simulink model "Team_Fire_Simulink_Model_Final_Presantation"  (R2025a)
settings: Solver=VariableStepAuto  StartTime=0.0  StopTime=12  RelTol=1e-3
libraries: spsControlledVoltageSourceLib x1, spsDCMachineLib x1, fl_lib x1, simulink x1, SignalEditorBlockLib x1, sps_lib x1
settings Model: Creator=Naresh Tuppathi  LastModifiedBy=berka

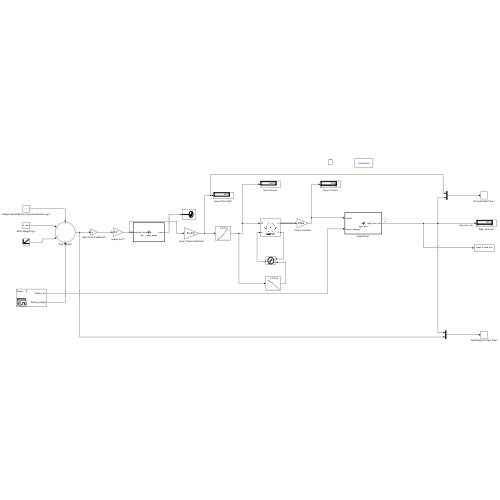
[thumbnail: Simulink's stored preview of the top-level diagram]
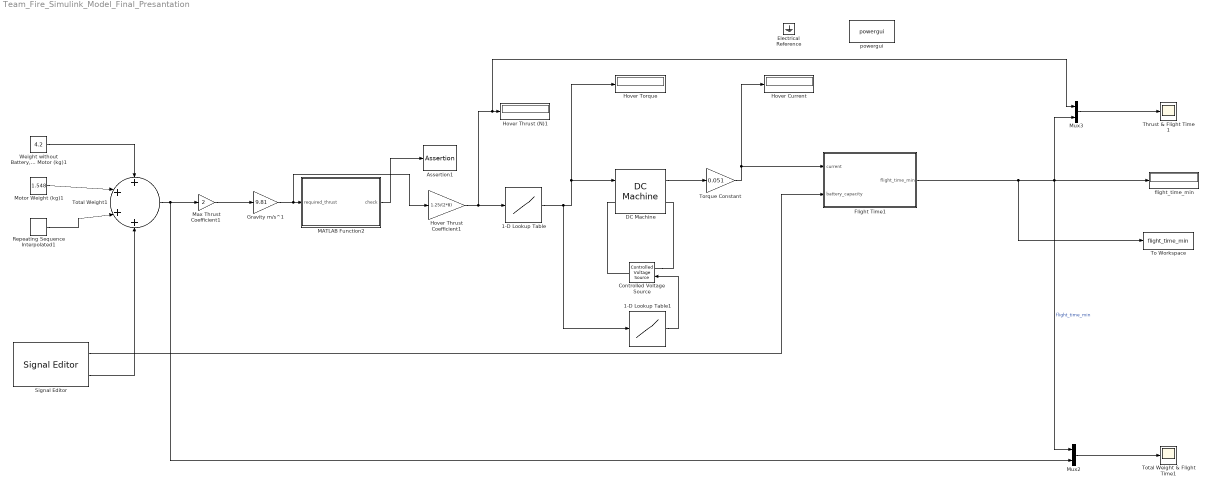
== system Team_Fire_Simulink_Model_Final_Presantation ==
  1-D Lookup Table : Lookup_n-D  NumberOfTableDimensions=1  BreakpointsForDimension1=[13.2 14.1 15.2 16.1 17.2 18.4 19.6 20.7 21.8 23.1 24.1 25.3 26.5 28.0 29.5 30.6 36.8 38.1 42.6 50.1]  Table=[0.30 0.32 0.34 0.36 0.39 0.41 0.43 0.46 0.48 0.51 0.53 0.56 0.59 0.62 0.65 0.67 0.96 0.98 1.04 1.10]  InternalRulePriority=Speed  RndMeth=Simplest
  1-D Lookup Table1 : Lookup_n-D  NumberOfTableDimensions=1  BreakpointsForDimension1=[0.30 0.32 0.34 0.36 0.39 0.41 0.43 0.46 0.48 0.51 0.53 0.56 0.59 0.62 0.65 0.67 0.80 0.94 1.10]  Table=[24.32 24.31 24.29 24.28 24.27 24.26 24.25 24.24 24.22 24.21 24.20 24.19 24.17 24.15 24.13 24.11 24.03 23.94 23.80]  InternalRulePriority=Speed  RndMeth=Simplest
  Assertion1 : Assertion
  Controlled Voltage Source : spsControlledVoltageSourceLib/Controlled Voltage Source  Initialize=on  Source_Type=DC  Amplitude=24  Phase=0  Frequency=0  Measurements=None
  DC Machine : spsDCMachineLib/DC Machine  PresetModel=No  MechanicalLoad=Torque TL  FieldType=Permanent magnet  ShowDetailedParameters=on  MeasurementBus=off  RLa="[ 0.05  12^-6]"  RLf="[ 240  120]"  Laf=1.8  MachineConstant=Torque constant (N.m/A)  Ke=1.8  Kt=0.078  J=0.0001  Bm=10^-7  Tf=0.01  w0=0  Ifinit=1  TsPowergui=0  TsBlock=-1
  Electrical Reference : fl_lib/Electrical/Electrical Elements/Electrical Reference
  Flight Time1 : MATLAB Function  TreatAsAtomicUnit=on
  Gravity m/s^1 : Gain  Gain=9.81
  Hover Current : Display
  Hover Thrust (N)1 : Display
  Hover Thrust Coefficient1 : Gain  Gain=1.25/(2*8)
  Hover Torque : Display
  MATLAB Function2 : MATLAB Function  TreatAsAtomicUnit=on
  Max Thrust Coefficient1 : Gain  Gain=2
  Motor Weight (kg)1 : Constant  Value=1.548
  Mux2 : Mux  Inputs=2
  Mux3 : Mux  Inputs=2
  Repeating Sequence Interpolated1 : simulink/Sources/Repeating Sequence Interpolated  OutValues=[0 1.5 3 4.5 6 7.5 9].'  TimeValues=[0 2 4 6 8 10 12].'  LookUpMeth=Interpolation-Use End Values  tsamp=0.01  OutMin=[]  OutMax=[]  OutDataTypeStr=double  OutputDataTypeScalingMode=double  OutDataType=fixdt(0,8)  OutScaling=2^-10
  Signal Editor : SignalEditorBlockLib/Signal Editor  FileName=C:\Users\berka\OneDrive\Masaüstü\CHAM LECTURE\Case Study Mechatronic System Simulation\battery_scenarios.mat  ActiveScenario=battery_1  ActiveSignal=battery_ah  IsBus=off  OutputBusObjectStr=Bus: BusObject  SampleTime=0  ZeroCross=off  OutputAfterFinalValue=Setting to zero  Unit=inherit  PreserveSignalName=on  ApplySigPropsToAllScenarios=on  ApplySigPropsToAllSignals=on  SignalPropertySource=Dialog parameters
  Thrust & Flight Time 1 : Scope
      settings: ActiveDisplayYMinimum=-26.545794074887681  ActiveDisplayYMaximum=59.278188161924348  DataLoggingVariableName=ScopeData2
  To Workspace : ToWorkspace  VariableName=flight_time_min  SampleTime=-1
      settings: MaxDataPoints=Inf
  Torque Constant : Gain  Gain=0.051
  Total Weight & Flight Time1 : Scope
      settings: ActiveDisplayYMinimum=5.03764  ActiveDisplayYMaximum=64.14121  DataLoggingVariableName=ScopeData3
  Total Weight1 : Sum  Inputs=++++
  "Weight without Battery, Payload and Motor (kg)1" : Constant  Value=4.2
  flight_time_min : Display
  powergui : sps_lib/powergui  Priority=1  SimulationMode=Continuous  SampleTime=50e-6  frequency=60  Iterations=50  frequencyindice=0  Pbase=100e6  ErrMax=1e-4  UnitsV=kV  UnitsW=MW  buscounter=0  FunctionMessages=off  echomessages=off  EnableUseOfTLC=off  CurrentSourceSwitches=off  DisableSnubberDevices=off  DisableRonSwitches=off  DisableVfSwitches=off  DisplayEquations=off  AutomaticDiscreteSolvers=off  SolverType=Tustin/Backward Euler (TBE)  Interpol=off  ExternalGateDelay=off  methode=off  Ts=100  x0status=blocks  SPID=on  SwTol=0  HookPort=off  NonlinearTolerance=1e-4  nMaxIteration=100  ContinueOnMaxIteration=off  RestoreLinks=warning  ResistiveCurrentMeasurement=off  Frange=[0:2:500]  Ylog=off  Xlog=on  ShowGrid=off  save=off  variable=ZData  structure=0  ZoomFFT=off  StartTime=0.0  cycles=1  DisplayStyle=1  fundamental=60  FreqAxis=off  MaxFrequency=1000  frequencyindicesteady=1  RmsSteady=1  display=off
  wires:
  Mux3/1 -> Thrust & Flight Time 1/1
  Repeating Sequence Interpolated1/1 -> Total Weight1/3
  Flight Time1/1(flight_time_min) -> flight_time_min/1, Mux2/1, Mux3/2, To Workspace/1  "flight_time_min"
  Total Weight1/1 -> Max Thrust Coefficient1/1, Mux2/2
  MATLAB Function2/1(check) -> Assertion1/1
  Mux2/1 -> Total Weight & Flight Time1/1
  Motor Weight (kg)1/1 -> Total Weight1/2
  Gravity m/s^1/1 -> Hover Thrust Coefficient1/1, MATLAB Function2/1(required_thrust)
  "Weight without Battery, Payload and Motor (kg)1"/1 -> Total Weight1/1
  1-D Lookup Table/1 -> 1-D Lookup Table1/1, Hover Torque/1, DC Machine/1
  Max Thrust Coefficient1/1 -> Gravity m/s^1/1
  Hover Thrust Coefficient1/1 -> Hover Thrust (N)1/1, Mux3/1, 1-D Lookup Table/1
  DC Machine/1 -> Torque Constant/1
  Torque Constant/1 -> Hover Current/1, Flight Time1/1(current)
  Signal Editor/2 -> Total Weight1/4
  Signal Editor/1 -> Flight Time1/2(battery_capacity)
  1-D Lookup Table1/1 -> Controlled Voltage Source/1
  connections:
  Controlled Voltage Source/RConn1 -- DC Machine/LConn1
  Controlled Voltage Source/LConn1 -- DC Machine/RConn1

== matlab function Team_Fire_Simulink_Model_Final_Presantation/MATLAB Function2 ==
  data: required_thrust input; check output
function check = maxThrustCheck(required_thrust)
    % INPUT: required_thrust (N) from Simulink
    max_thrust_per_motor = 54.4;  % N
    num_motors = 8;
    max_total_thrust = max_thrust_per_motor * num_motors;
    check = (required_thrust <= max_total_thrust);
end

== matlab function Team_Fire_Simulink_Model_Final_Presantation/Flight Time1 ==
  data: current input; flight_time_min output; battery_capacity input
function flight_time_min = FlightTime(current, battery_capacity)
    % INPUTS:
    %   current [A]             : motor başına akım
    %   battery_capacity [Ah]   : toplam batarya kapasitesi (örneğin 60 Ah)

    current = double(current);
    battery_capacity = double(battery_capacity);

    % Toplam akım [A]
    total_current = current * 8;

    % Süre [saat] = kapasite / toplam akım
    time_hr = battery_capacity / total_current;

    % Süre [dakika]
    time_min = time_hr * 60;

    % %15 güvenlik payı ile gerçek uçuş süresi
    flight_time_min = time_min * 0.85;
end
